simulink model "smib_milano6ord"  (R2022b)
settings: Solver=VariableStepAuto  StartTime=0.0  StopTime=10.0  RelTol=1e-3
settings Model: Creator=jmmau  LastModifiedBy=jmmau

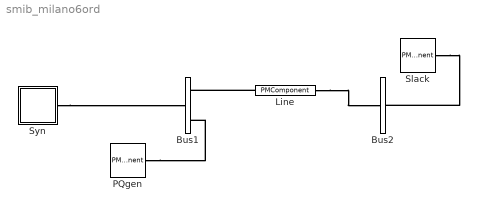
== system smib_milano6ord ==
  Bus1 : PMComponent  Tag=PSATblock  Description=Connection  PhysicalDomain=psatdomain  LeftPortType=p1  RightPortType=p1  LConnTagsString=__newl0|__newl1  RConnTagsString=__newr0  mask(Bus){in=2, out=1, p2q=20, p3_4q=[1.00  0.00], p5q=1, p6q=1}
      mask prompts: in "Number of inputs:"; out "Number of outputs:"; p2q "Voltage Rating [kV]"; p3_4q "Voltage initial guess [p.u.  rad]"; p5q "Area number"; p6q "Region number"
      mask help: Bus block.
      mask init:
      | fm_inout
      mask Callback p5q: fm_block
      mask Display: plot([0 1 1 0 0],[0 0 1 1 0])
  Bus2 : PMComponent  Tag=PSATblock  Description=Connection  PhysicalDomain=psatdomain  LeftPortType=p1  RightPortType=p1  LConnTagsString=__newl0  RConnTagsString=__newr0  mask(Bus){in=1, out=1, p2q=20, p3_4q=[1.00  0.00], p5q=1, p6q=1}
      mask prompts: in "Number of inputs:"; out "Number of outputs:"; p2q "Voltage Rating [kV]"; p3_4q "Voltage initial guess [p.u.  rad]"; p5q "Area number"; p6q "Region number"
      mask help: Bus block.
      mask init:
      | fm_inout
      mask Callback p5q: fm_block
      mask Display: plot([0 1 1 0 0],[0 0 1 1 0])
  Line : PMComponent  Tag=PSATblock  Description=Power Flow  PhysicalDomain=psatdomain  LeftPortType=p1  RightPortType=p1  LConnTagsString=__newl0  RConnTagsString=__newr0  mask(Line){p3_4_5q=[200e3  20  50], p6q=0, p8q=0.01, p9q=0.05, p10q=0, p13_14_15q=[0.0  0.0  0.0], p16q=on}
      mask prompts: p3_4_5q "Power, Voltage and Frequency Ratings [MVA, kV, Hz]"; p6q "Length of line [km] (0 for p.u. parameters)"; p8q "Resistance [p.u. (Ohms/km)]"; p9q "Reactance [p.u. (H/km)]"; p10q "Susceptance [p.u. (F/km)]"; p13_14_15q "Imax, Pmax and Smax [p.u., p.u., p.u.]"; p16q "Connected"
      mask help: This block defines a pi model for a tree phase line.
      mask init:
      | [xp,yp] = fm_draw('pi');
      mask Callback p16q: fm_block
      mask Display:
      | plot([-1  1  1 -1 -1],[-0.2 -0.2 0.2 0.2 -0.2])
      | color('blue')
      | plot(0.35*xp,0.2*yp)
  PQgen : PMComponent  Tag=PSATblock  Description=Power Flow  PhysicalDomain=psatdomain  LeftPortType=p1  RightPortType=p1  RConnTagsString=__newr0  mask(PQgen){p2_3q=[1500  20], p4_5q=[0.8  0.6], p6_7q=[1.1  0.9], p8q=off, p9q=on}
      mask prompts: p2_3q "Power and Voltage Ratings [MVA, kV]"; p4_5q "Active and Reactive Powers [p.u.  p.u.]"; p6_7q "Vmax and Vmin [p.u.  p.u.]"; p8q "Allow conversion to impedance"; p9q "Connected"
      mask help: This block defines a PQ generator.
      mask init:
      | [x,y] = fm_draw('circle');
      | [xp,yp] = fm_draw('P');
      | [xq,yq] = fm_draw('Q');
      mask Callback p8q: fm_block
      mask Callback p9q: fm_block
      mask Display:
      | plot(x,y)
      | color('blue')
      | plot(0.3*xp-0.35,0.6*yp,0.4*xq+0.1,0.6*yq)
  Slack : PMComponent  Tag=PSATblock  Description=Power Flow  PhysicalDomain=psatdomain  LeftPortType=p1  RightPortType=p1  RConnTagsString=__newr0  mask(SW){p2_3q=[2000  20], p4q=1.00, p5q=0.00, p6_7q=[1.5  -1.5], p8_9q=[1.1  0.9], p10q=0.80, p11q=1, p12q=on, p13q=on}
      mask prompts: p2_3q "Power and Voltage Ratings [MVA, kV]"; p4q "Voltage Magnitude [p.u.]"; p5q "Reference Phase Angle [rad]"; p6_7q "Qmax and Qmin [p.u.  p.u.]"; p8_9q "Vmax and Vmin  [p.u.  p.u.]"; p10q "Active Power Guess [p.u.]"; p11q "Loss Participation Factor"; p12q "Reference bus"; p13q "Connected"
      mask help:
      | This block defines a V-theta bus:
      |
      | V = V_des
      | theta = theta_des
      mask init:
      | [x,y] = fm_draw('circle');
      | [xt,yt] = fm_draw('theta');
      mask Callback p12q: fm_block
      mask Callback p13q: fm_block
      mask Display: plot([0 1 1 0 0],[0 0 1 1 0]), color('blue'), plot([0 1],[0 1],[0 1],[1 0],[0.5 1 0.5 0 0.5],[0 0.5 1 0.5 0])
  Syn : Subsystem  Tag=PSATblock  Description=Machines  mask(Syn){p2_3_4q=[1500  20   50], p5q=6, p7_6q=[0.0  0.234], p8_9_10q=[2.135  0.34  0.269], p11_12q=[6.47  0.022], p13_14_15q=[2.046  0.573  0.269], p16_17q=[0.61  0.034], p18_19q=[2*6.3  0.00], p20_21q=[0.00  0.00], p22_23q=[1.00  1.00], p24q=0.0, p25_26q=[0 0], in=0, p27q=1, p28q=on}
      mask prompts: p2_3_4q "Power, voltage and frequency ratings [MVA, kV, Hz]"; p5q "Machine Dynamic Order"; p7_6q "resistance ra and leakage reactance xl [p.u. p.u.]"; p8_9_10q "d-axis reactances Xd, X'd X"d [p.u.,p.u.,p.u.]"; p11_12q "d-axis open circuit time constants T'd0 and T"d0 [s, s]"; p13_14_15q "q-axis reactances Xq, X'q, X"q [p.u.  p.u.  p.u.]"; p16_17q "q-axis open circuit time constants T'q0 and T"q0 [s s]"; p18_19q "Inertia (M = 2H) and Damping [s, p.u.]"; p20_21q "Speed and active power additional signals Kw and Kp [p.u., p.u.]"; p22_23q "Percentage of active and reactive powers at bus [p.u. p.u.]"; p24q "d-axis additional circuit leakage time constant Taa [s]"; p25_26q "Saturation coefficients S(1.0) and S(1.2)"; in "Number of input signals"; p27q "COI number"; p28q "Connected"
      mask help: This block defines a fourth order synchronous machine.
      mask init:
      | fm_inout
      | [x,y] = fm_draw('circle');
      | [xg,yg] = fm_draw('G');
      | [xs,ys] = fm_draw('sinus');
      mask TypeOptions p5q: 8 | 6 | 5.3 | 5.2 | 5.1 | 4 | 3 | 2
      mask Callback p5q: fm_block
      mask TypeOptions in: 0 | 1 | 2
      mask Callback p28q: fm_block
      mask Display:
      | plot(x+1.4,y,0.12*xs+1,0.15*ys-0.6)
      | color('blue')
      | plot(1.4+0.45*xg,0.3+0.45*yg)
  connections:
  Syn/RConn1 -- Bus1/RConn1
  Slack/RConn1 -- Bus2/LConn1
  PQgen/RConn1 -- Bus1/LConn2
  Line/LConn1 -- Bus1/LConn1
  Line/RConn1 -- Bus2/RConn1

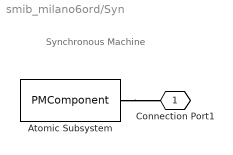
== system smib_milano6ord/Syn ==
  note: Synchronous Machine
  Atomic Subsystem : PMComponent  PhysicalDomain=psatdomain  LeftPortType=p1  RightPortType=p1  RConnTagsString=__newr0
  Connection Port1 : PMIOPort  Tag=PMCPort  Side=Right
  connections:
  Atomic Subsystem/RConn1 -- Connection Port1/RConn1
